simulink subsystem "AD7173_8_ADC"  (R2022b)
settings: Solver=VariableStepAuto  StartTime=0.0  StopTime=10.0  RelTol=1e-3
values from neighbouring files (symbols this model uses):
  AD7173_8_INIT = bitconcat(ufi(AD7173_8_INIT_tmp(:,1),8,0),ufi(AD7173_8_INIT_tmp(:,2),16,0))    [init_SYSTEM.m]
libraries: hdlsllib x7, simulink x7
Description:
  | Copyright (c) 2023, Alexei Evsenin, evsenin@gmail.com
settings Model: Creator=evsenin  LastModifiedBy=evsenin
settings ModelReferenceCC: EnableRefExpFcnMdlSchedulingChecks=on

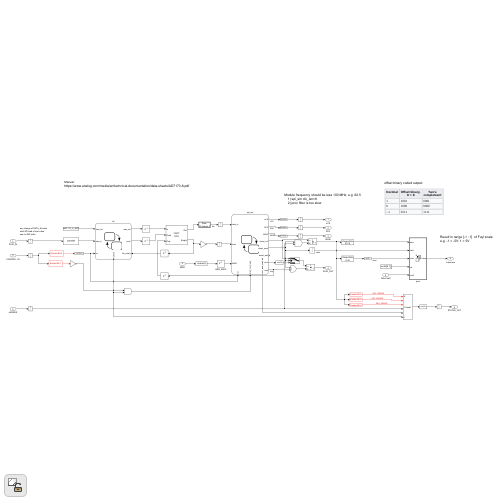
[thumbnail: Simulink's stored preview of the top-level diagram]
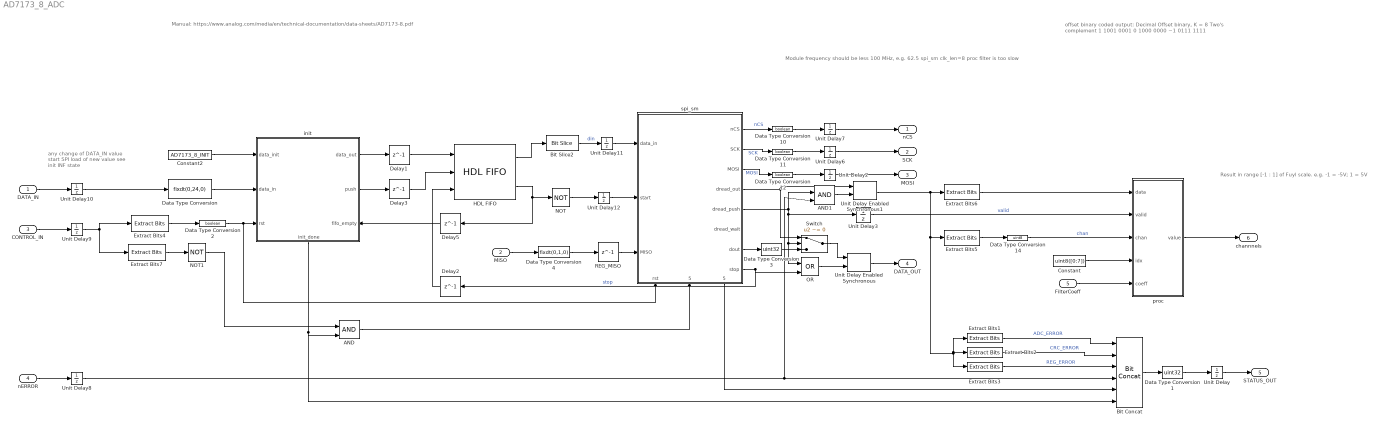
== system AD7173_8_ADC ==
  note: any change of DATA_IN value
      | start SPI load of new value
      | see init INF state
  note: Module frequency should be less 100 MHz, e.g. 62.5
      | spi_sm clk_len=8
      | proc filter is too slow
  note: Manual:
      | https://www.analog.com/media/en/technical-documentation/data-sheets/AD7173-8.pdf
  note: offset binary coded output:
      |
      | Decimal
      | Offset binary,
      | K = 8
      | Two's
      | complement
      |
      | 1
      | 1001
      | 0001
      |
      | 0
      | 1000
      | 0000
      |
      | −1
      | 0111
      | 1111
  note: Result in range [-1 : 1] of Fuyl scale.
      | e.g. -1 = -5V; 1 = 5V
  DATA_IN : Inport
  MISO : Inport  Port=2
  CONTROL_IN : Inport  Port=3
  nERROR : Inport  Port=4
  FilterCoeff : Inport  Port=5
  AND : Logic  IconShape=distinctive  AllPortsSameDT=off  OutDataTypeStr=boolean
  AND1 : Logic  IconShape=distinctive  AllPortsSameDT=off  OutDataTypeStr=boolean
  Bit Concat : hdlsllib/Logic and Bit Operations/Bit Concat  numInputs=6
  Bit Slice2 : hdlsllib/Logic and Bit Operations/Bit Slice  lidx=23  ridx=0
  Constant : Constant  Value=uint8([0:7])  SampleTime=-1
  Constant2 : Constant  Value=AD7173_8_INIT  OutDataTypeStr=fixdt(0,24,0)  SampleTime=-1
  Data Type Conversion : DataTypeConversion  OutDataTypeStr=fixdt(0,24,0)  SaturateOnIntegerOverflow=off  RndMeth=Floor
  Data Type Conversion1 : DataTypeConversion  OutDataTypeStr=uint32  SaturateOnIntegerOverflow=off  RndMeth=Floor
  Data Type Conversion{2,10..12} (4 alike) : DataTypeConversion  OutDataTypeStr=boolean  SaturateOnIntegerOverflow=off  RndMeth=Floor
  Data Type Conversion14 : DataTypeConversion  OutDataTypeStr=uint8  SaturateOnIntegerOverflow=off  RndMeth=Floor
  Data Type Conversion3 : DataTypeConversion  OutDataTypeStr=uint32  SaturateOnIntegerOverflow=off  RndMeth=Floor
  Data Type Conversion4 : DataTypeConversion  OutDataTypeStr=fixdt(0,1,0)  SaturateOnIntegerOverflow=off  RndMeth=Floor
  Delay{1..3,5} (4 alike) : Delay  DelayLength=1
  Extract Bits1 : simulink/Logic and Bit Operations/Extract Bits  bitsToExtract=Range of bits  numBits=8  bitIdxRange=6  outScalingMode=Treat bit field as an integer
  Extract Bits2 : simulink/Logic and Bit Operations/Extract Bits  bitsToExtract=Range of bits  numBits=8  bitIdxRange=5  outScalingMode=Treat bit field as an integer
  Extract Bits3 : simulink/Logic and Bit Operations/Extract Bits  bitsToExtract=Range of bits  numBits=8  bitIdxRange=4  outScalingMode=Treat bit field as an integer
  Extract Bits4 : simulink/Logic and Bit Operations/Extract Bits  bitsToExtract=Range of bits  numBits=8  bitIdxRange=0  outScalingMode=Treat bit field as an integer
  Extract Bits5 : simulink/Logic and Bit Operations/Extract Bits  bitsToExtract=Range of bits  numBits=8  bitIdxRange=[0 3]  outScalingMode=Treat bit field as an integer
  Extract Bits6 : simulink/Logic and Bit Operations/Extract Bits  bitsToExtract=Range of bits  numBits=8  bitIdxRange=[8 31]  outScalingMode=Treat bit field as an integer
  Extract Bits7 : simulink/Logic and Bit Operations/Extract Bits  bitsToExtract=Range of bits  numBits=8  bitIdxRange=1  outScalingMode=Treat bit field as an integer
  HDL FIFO : hdlsllib/HDL RAMs/HDL FIFO  fifo_size=64  mode=FWFT  ratio=1  push_msg=Warning  pop_msg=Warning  show_empty=on  show_full=off  show_num=off  LabelModeActiveChoice_Mode=FWFT  rst_port=off
  NOT : Logic  Operator=NOT  IconShape=distinctive  AllPortsSameDT=off  OutDataTypeStr=boolean
  NOT1 : Logic  Operator=NOT  IconShape=distinctive  AllPortsSameDT=off  OutDataTypeStr=boolean
  OR : Logic  Operator=OR  IconShape=distinctive  AllPortsSameDT=off  OutDataTypeStr=boolean
  REG_MISO : Delay  DelayLength=1
  Switch : Switch  Criteria=u2 ~= 0  SaturateOnIntegerOverflow=off  InputSameDT=off
  Unit Delay{,2..3,6..12} (10 alike) : UnitDelay  SampleTime=-1  HasFrameUpgradeWarning=on
  Unit Delay Enabled Synchronous : hdlsllib/Discrete/Unit Delay Enabled Synchronous  InitialCondition=0.0  SampleTime=-1
  Unit Delay Enabled Synchronous1 : hdlsllib/Discrete/Unit Delay Enabled Synchronous  InitialCondition=0.0  SampleTime=-1
  init : Stateflow chart  TreatAsAtomicUnit=on
      settings: PortSchema="{\"entries\":[{\"content\":{\"sides\":[{\"content\":{\"connectorIds\":[\"In1\",\"In2\",\"In4\"]},\"type\":\"ConnectorPlacement.EquallySpacedRectSide\",\"uuid\":\"2541893e-0497-4685-a403-0c18c6ba8828\"},{\"content\":{\"connectorIds\":[\"Out2\",\"Out1\",\"In3\"],\"side\":\"RIGHT\"},\"type\":\"ConnectorPlacement.EquallySpacedRectSide\",\"uuid\":\"ea7d69d9-7294-4ef3-b4a5-e03a3485fcd1\"},{\"content\":{\"connectorIds\":[],\"side\":\"TOP\"},\"type\":\"ConnectorPlacement.EquallySpacedRectSide\",\"uuid\":\"4588f9c3-6d00-4467-b78c-e50bd35827d1\"},{\"content\":{\"connectorIds\":[\"Out3\"],\"side\":\"BOTTOM\"},\"type\":\"ConnectorPlacement.EquallySpacedRectSide\",\"uuid\":\"6cf1debc-d261-40b7-9985-8c0ec2d9837a\"},{\"content\":{\"connectorIds\":[],\"side\":\"HIDDEN\"},\"type\":\"ConnectorPlacement.EquallySpacedRectSide\",\"uuid\":\"32712179-057e-4c85-bea4-acb9bd43153e\"}]},\"type\":\"ConnectorPlacement.EquallySpacedConnector\",\"uuid\":\"4c1de655-9fa7-4102-a0fe-e6132f80d46b\"}],\"packageUris\":[\"http://schema.mathworks.com/mf0/Connector/R2020b\"],\"version\":\"1.0\"}"
  proc : Subsystem  TreatAsAtomicUnit=on
  spi_sm : Stateflow chart  TreatAsAtomicUnit=on
      settings: PortSchema="{\"entries\":[{\"content\":{\"sides\":[{\"content\":{\"connectorIds\":[\"In1\",\"In3\",\"In2\"]},\"type\":\"ConnectorPlacement.EquallySpacedRectSide\",\"uuid\":\"c873ee2d-afd2-4da8-a43b-135f6a354a0c\"},{\"content\":{\"connectorIds\":[\"Out1\",\"Out3\",\"Out2\",\"Out7\",\"Out6\",\"Out9\",\"Out8\",\"Out4\"],\"side\":\"RIGHT\"},\"type\":\"ConnectorPlacement.EquallySpacedRectSide\",\"uuid\":\"424a6b82-da04-4858-9164-e360fe3abeb3\"},{\"content\":{\"connectorIds\":[],\"side\":\"TOP\"},\"type\":\"ConnectorPlacement.EquallySpacedRectSide\",\"uuid\":\"9ec86d72-b4ed-4894-a0c0-a4fac65a3c4c\"},{\"content\":{\"connectorIds\":[\"In4\",\"In5\",\"Out5\"],\"side\":\"BOTTOM\"},\"type\":\"ConnectorPlacement.EquallySpacedRectSide\",\"uuid\":\"9ef91c08-c58e-42aa-944d-546a3b799edc\"},{\"content\":{\"connectorIds\":[],\"side\":\"HIDDEN\"},\"type\":\"ConnectorPlacement.EquallySpacedRectSide\",\"uuid\":\"d113467b-580b-4249-84bc-ee2c7951f3a5\"}]},\"type\":\"ConnectorPlacement.EquallySpacedConnector\",\"uuid\":\"111a2709-fa96-4e2c-b71d-d73d8b96bd37\"}],\"packageUris\":[\"http://schema.mathworks.com/mf0/Connector/R2020b\"],\"version\":\"1.0\"}"
  nCS : Outport
  SCK : Outport  Port=2
  MOSI : Outport  Port=3
  DATA_OUT : Outport  Port=4
  STATUS_OUT : Outport  Port=5
  channnels : Outport  Port=6
  wires:
  Data Type Conversion4/1 -> REG_MISO/1
  Bit Slice2/1 -> Unit Delay11/1  "din"
  MISO/1 -> Data Type Conversion4/1
  spi_sm/3(SCK) -> Data Type Conversion11/1  "SCK"
  spi_sm/2(MOSI) -> Data Type Conversion12/1  "MOSI"
  spi_sm/4(stop) -> OR/2, Delay2/1  "stop"
  HDL FIFO/1 -> Bit Slice2/1
  HDL FIFO/2 -> NOT/1, Delay5/1
  NOT/1 -> Unit Delay12/1
  Delay2/1 -> HDL FIFO/3
  init/1(push) -> Delay3/1
  init/2(data_out) -> Delay1/1
  DATA_IN/1 -> Unit Delay10/1
  Data Type Conversion/1 -> init/2(data_in)
  Data Type Conversion3/1 -> Switch/3
  spi_sm/1(nCS) -> Data Type Conversion10/1  "nCS"
  Constant2/1 -> init/1(data_init)
  CONTROL_IN/1 -> Unit Delay9/1
  REG_MISO/1 -> spi_sm/2(MISO)
  init/3(init_done) -> AND/2, Bit Concat/6
  Delay1/1 -> HDL FIFO/1
  Delay3/1 -> HDL FIFO/2
  Delay5/1 -> init/3(fifo_empty)
  Extract Bits4/1 -> Data Type Conversion2/1
  spi_sm/6(dread_push) -> Unit Delay3/1, Switch/2, OR/1, AND1/1
  spi_sm/8(dout) -> Data Type Conversion3/1
  Bit Concat/1 -> Data Type Conversion1/1
  nERROR/1 -> Unit Delay8/1
  Data Type Conversion1/1 -> Unit Delay/1
  Unit Delay/1 -> STATUS_OUT/1
  Unit Delay2/1 -> MOSI/1
  Unit Delay3/1 -> proc/2(valid)  "valid"
  Unit Delay Enabled Synchronous1/1 -> Extract Bits6/1, Extract Bits5/1, Extract Bits3/1, Extract Bits2/1, Extract Bits1/1
  Unit Delay6/1 -> SCK/1
  Unit Delay7/1 -> nCS/1
  Unit Delay9/1 -> Extract Bits4/1, Extract Bits7/1
  Unit Delay10/1 -> Data Type Conversion/1
  Unit Delay11/1 -> spi_sm/1(data_in)
  Unit Delay12/1 -> spi_sm/3(start)
  spi_sm/7(dread_out) -> Unit Delay Enabled Synchronous1/1, Switch/1
  Extract Bits1/1 -> Bit Concat/1  "ADC_ERROR"
  Extract Bits2/1 -> Bit Concat/2  "CRC_ERROR"
  Extract Bits3/1 -> Bit Concat/3  "REG_ERROR"
  Data Type Conversion10/1 -> Unit Delay7/1
  Data Type Conversion11/1 -> Unit Delay6/1
  Data Type Conversion12/1 -> Unit Delay2/1
  Extract Bits5/1 -> Data Type Conversion14/1
  Data Type Conversion14/1 -> proc/3(chan)  "chan"
  Extract Bits6/1 -> proc/1(data)
  Constant/1 -> proc/4(idx)
  proc/1(value) -> channnels/1
  FilterCoeff/1 -> proc/5(coeff)
  Extract Bits7/1 -> NOT1/1
  AND/1 -> spi_sm/5(start_cont_read)
  NOT1/1 -> AND/1
  Data Type Conversion2/1 -> init/4(rst), spi_sm/4(rst)
  OR/1 -> Unit Delay Enabled Synchronous/2
  Unit Delay Enabled Synchronous/1 -> DATA_OUT/1
  Unit Delay8/1 -> Bit Concat/4, AND1/2
  spi_sm/5(cont_read_enabled) -> Bit Concat/5
  Switch/1 -> Unit Delay Enabled Synchronous/1
  AND1/1 -> Unit Delay Enabled Synchronous1/2

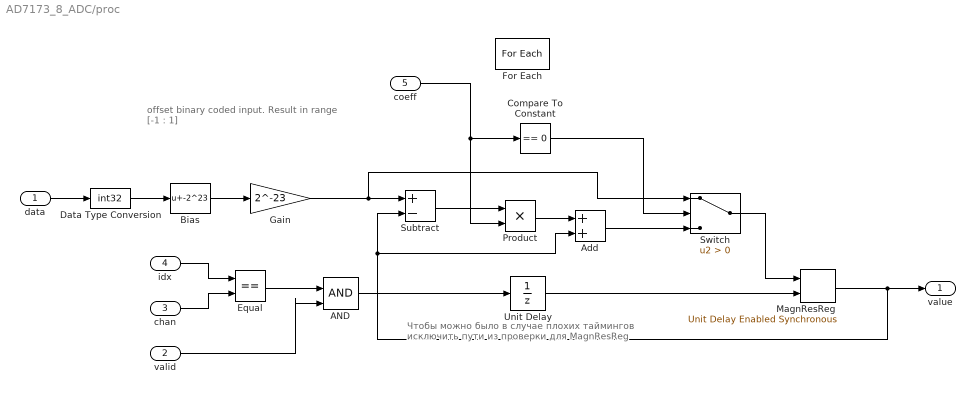
== system AD7173_8_ADC/proc ==
  note: Чтобы можно было в случае плохих таймингов
      | исключить пути из проверки для MagnResReg
  note: offset binary coded input.
      | Result in range [-1 : 1]
  data : Inport
  valid : Inport  Port=2
  chan : Inport  Port=3
  idx : Inport  Port=4  Partition=on  PartitionDimension=1  PartitionWidth=1  PartitionOffset=0
  coeff : Inport  Port=5
  AND : Logic  IconShape=distinctive  AllPortsSameDT=off  OutDataTypeStr=boolean
  Add : Sum  SaturateOnIntegerOverflow=on  OutDataTypeStr=Inherit: Same as first input
  Bias : Bias  Bias=-2^23
  Compare To Constant : hdlsllib/Logic and Bit Operations/Compare To Constant  relop===  const=0  OutDataTypeStr=boolean
  Data Type Conversion : DataTypeConversion  OutDataTypeStr=int32  SaturateOnIntegerOverflow=off  RndMeth=Floor
  Equal : RelationalOperator  Operator===  OutDataTypeStr=boolean  RndMeth=Simplest  InputSameDT=off
  For Each : ForEach  DisableCoverage=on
  Gain : Gain  Gain=2^-23  OutDataTypeStr=fixdt(1,32,31)  SaturateOnIntegerOverflow=on
  MagnResReg : hdlsllib/Discrete/Unit Delay Enabled Synchronous  InitialCondition=0.0  SampleTime=-1
  Product : Product  SaturateOnIntegerOverflow=on  OutDataTypeStr=Inherit: Same as first input
  Subtract : Sum  Inputs=+-  OutDataTypeStr=fixdt(1,32,31)  SaturateOnIntegerOverflow=on
  Switch : Switch  Criteria=u2 > Threshold  SaturateOnIntegerOverflow=off  InputSameDT=off
  Unit Delay : UnitDelay  SampleTime=-1  HasFrameUpgradeWarning=on
  value : Outport  ConcatenationDimension=1
  wires:
  Data Type Conversion/1 -> Bias/1
  Gain/1 -> Subtract/1, Switch/1
  Bias/1 -> Gain/1
  data/1 -> Data Type Conversion/1
  Switch/1 -> MagnResReg/1
  Add/1 -> Switch/3
  Compare To Constant/1 -> Switch/2
  Unit Delay/1 -> MagnResReg/2
  Product/1 -> Add/1
  coeff/1 -> Product/2, Compare To Constant/1
  Subtract/1 -> Product/1
  MagnResReg/1 -> Subtract/2, Add/2, value/1
  chan/1 -> Equal/2
  idx/1 -> Equal/1
  valid/1 -> AND/2
  Equal/1 -> AND/1
  AND/1 -> Unit Delay/1

== stateflow chart AD7173_8_ADC/spi_sm ==
  settings: executeAtInitialization=1
  state CONT_READ_GET
    en:
    nCS = 0;
    MOSI = 0;
    dread_out = 0;
    cnt_clk = clk_len;
    cnt_bit = 32;
    du:
    cnt_clk = cnt_clk - 1;
    if cnt_clk > bitshift(clk_len,-1)
    SCK = 0;
    else
    SCK = 1;
    end
    if cnt_clk == bitshift(clk_len,-1)
    dread_out = bitset(dread_out, cnt_bit, MISO);
    end
    if cnt_clk == 0
    cnt_clk = clk_len;
    cnt_bit = cnt_bit - 1;
    end
    if cnt_bit == 0
    dread_push = true;
    end
  state CONT_READ_INIT
    en:
    nCS = 0;
    din = AD7173_8_IFMODE;
    cnt_clk = clk_len;
    cnt_bit = bit_len;
    du:
    cnt_clk = cnt_clk - 1;
    din = din;
    if bitget(din,cnt_bit) == 1
    MOSI = 1;
    else
    MOSI = 0;
    end
    if cnt_clk > bitshift(clk_len,-1)
    SCK = 0;
    else
    SCK = 1;
    end
    if cnt_clk == 0
    cnt_clk = clk_len;
    cnt_bit = cnt_bit - 1;
    end
    ex:
    nCS = 0;
    MOSI = 0;
    cont_read_enabled = true;
  state CONT_READ_WAIT_nRDY
    en:
    nCS = 0;
    MOSI = 0;
    cnt_clk = clk_len;
    cnt_bit = 32;
    dread_push = false;
    dread_wait = true;
    ex:
    dread_wait = false;
  state SW_RESET
    en:
    nCS = 0;
    SCK = 1;
    MOSI = 1;
    cnt_clk = clk_len;
    cnt_bit = 64;
    du:
    cnt_clk = cnt_clk - 1;
    if cnt_clk > bitshift(clk_len,-1)
    SCK = 0;
    else
    SCK = 1;
    end
    if cnt_clk == 0
    cnt_clk = clk_len;
    cnt_bit = cnt_bit - 1;
    end
    ex:
    nCS = 1;
    SCK = 1;
    MOSI = 0;
  note: Dealy 500us before next command
  state RESET
    nCS = ufi(1,1,0);
    SCK = ufi(1,1,0);
    MOSI = ufi(0,1,0);
    cnt_clk = uint8(0);
    cnt_bit = uint8(0);
    dout = ufi(0,24,0);
    din = ufi(0,24,0);
    cont_read_enabled = false;
    dread_out = ufi(0,32,0);
    dread_push = false;
    dread_wait = true;
  state IDLE
    nCS = 1;
    SCK = 1;
    MOSI = 0;
    cnt_clk = clk_len;
    cnt_bit = bit_len;
    din = data_in;
    cont_read_enabled = false;
    dread_wait = true;
  state WAIT_READY
  state ONE_TRANSACTION
    en:
    nCS = 0;
    dout = 0;
    cnt_clk = clk_len;
    cnt_bit = bit_len;
    din = data_in;
    du:
    cnt_clk = cnt_clk - 1;
    din = din;
    if bitget(din,cnt_bit) == 1
    MOSI = 1;
    else
    MOSI = 0;
    end
    if cnt_clk > bitshift(clk_len,-1)
    SCK = 0;
    else
    SCK = 1;
    end
    dout = bitset(dout, cnt_bit, MISO);
    if cnt_clk == 0
    cnt_clk = clk_len;
    cnt_bit = cnt_bit - 1;
    end
    ex:
    nCS = 1;
  state WAIT_nRDY
    dread_push = false;
  state WAIT
    en:
    stop = true;
    du:
    stop = false;
  CONT_READ_WAIT_nRDY -> RESET [order 1] : [rst]
  CONT_READ_INIT -> CONT_READ_WAIT_nRDY : [cnt_bit==0]
  CONT_READ_WAIT_nRDY -> CONT_READ_GET [order 2] : [MISO == 0]
  IDLE -> CONT_READ_INIT [order 3] : [start_cont_read]
  (default) -> RESET
  WAIT_nRDY -> CONT_READ_WAIT_nRDY [order 2] : after(clk_len,tick)[MISO == 1]
  CONT_READ_GET -> WAIT_nRDY : [dread_push]
  WAIT_READY -> IDLE : after(128*512,tick)
  SW_RESET -> WAIT_READY : [cnt_bit == 0]
  RESET -> SW_RESET : after(64,tick)[~rst]
  IDLE -> ONE_TRANSACTION [order 2] : [start]
  WAIT_nRDY -> RESET [order 1] : [rst]
  IDLE -> RESET [order 1] : [rst]
  WAIT -> IDLE : after(clk_len,tick)
  ONE_TRANSACTION -> WAIT : [cnt_bit == 0]
  data: data_in input fixdt(0,24,0); nCS output fixdt(0,1,0); MOSI output fixdt(0,1,0); cnt_clk local uint8; cnt_bit local uint8; MISO input fixdt(0,1,0); din local fixdt(0,24,0); SCK output fixdt(0,1,0); bit_len constant uint8 =24; clk_len constant uint8 =8; start input boolean; stop output boolean; rst input boolean; start_cont_read input boolean; cont_read_enabled output boolean; dread_push output boolean; dread_out output fixdt(0,32,0); dout output fixdt(0,24,0); AD7173_8_IFMODE parameter fixdt(0,24,0); dread_wait output

== stateflow chart AD7173_8_ADC/init ==
  settings: executeAtInitialization=1
  state INIT
    en:
    init_cnt = 0;
    push = false;
    init_done = false;
    du:
    if fifo_empty
    push = true;
    init_cnt = init_cnt + 1;
    data_out = data_init(init_cnt);
    else
    push = false;
    end
    ex:
    push = false;
  state RESET
    data_out = ufi(0,24,0);
    init_cnt = uint16(0);
    init_sz = uint16(length(data_init));
    push = false;
    data_in_prev = ufi(0,24,0);
    init_done = false;
  state WAIT0
  state INF
    en:
    data_in_prev = data_in;
    push = false;
    du:
    if data_in_prev ~= data_in
    push = true;
    else
    push = false;
    end
    data_in_prev = data_in;
    data_out = data_in;
    ex:
    push = false;
  state INIT_DONE
    init_done = true;
  (default) -> RESET
  INIT -> WAIT0 : [init_cnt == init_sz]
  RESET -> INIT : [~rst]
  WAIT0 -> INIT_DONE : [fifo_empty]
  INF -> RESET : [rst]
  INIT_DONE -> INF
  data: data_init input fixdt(0,24,0); push output boolean; init_cnt local uint16; data_out output fixdt(0,24,0); data_in input fixdt(0,24,0); data_in_prev local fixdt(0,24,0); init_sz local uint16; fifo_empty input boolean; init_done output boolean; rst input boolean
